simulink model "DiscCruiseController"  (Simulink 7.7)
settings: Solver=ode45  StartTime=0.0  StopTime=10.0  RelTol=1e-3
undefined symbols (not defined in the file): DT_Integrator, H, PID, suspension_lib, z
settings Model: Creator=jporter  LastModifiedBy=jporter

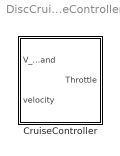
== system DiscCruiseController ==
  CruiseController : Subsystem

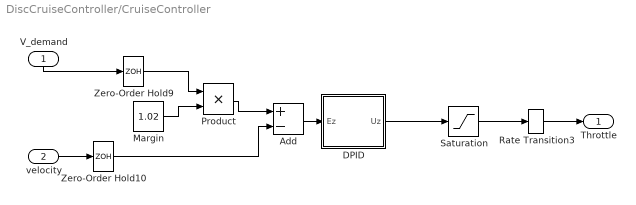
== system DiscCruiseController/CruiseController ==
  V_demand : Inport
  velocity : Inport  Port=2
  Add : Sum  Inputs=+-
  DPID : Subsystem  AncestorBlock=suspension_lib/PID:H(z)  mask{Ts=.1, K_P=7, K_D=0, tau_D=.1/pi, P_MAX=1500*2, P_MIN=-1500*2, X_DMAX=1500*2, X_DMIN=-1500*2, X_D0=0, K_I=0, X_IMAX=1500, X_IMIN=-1500, X_I0=0}
      mask prompts: Ts "Ts (seconds)"
  Margin : Constant  Value=1.02
  Product : Product  RndMeth=Zero
  Rate Transition3 : RateTransition  X0=1  OutPortSampleTime=0
  Saturation : Saturate  UpperLimit=1  LowerLimit=0
  Zero-Order Hold10 : ZeroOrderHold  Priority=-1  SampleTime=0.1
  Zero-Order Hold9 : ZeroOrderHold  Priority=-1  SampleTime=0.1
  Throttle : Outport
  wires:
  Product/1 -> Add/1
  Add/1 -> DPID/1(Ez)
  DPID/1(Uz) -> Saturation/1
  V_demand/1 -> Zero-Order Hold9/1
  velocity/1 -> Zero-Order Hold10/1
  Saturation/1 -> Rate Transition3/1
  Margin/1 -> Product/2
  Rate Transition3/1 -> Throttle/1
  Zero-Order Hold9/1 -> Product/1
  Zero-Order Hold10/1 -> Add/2

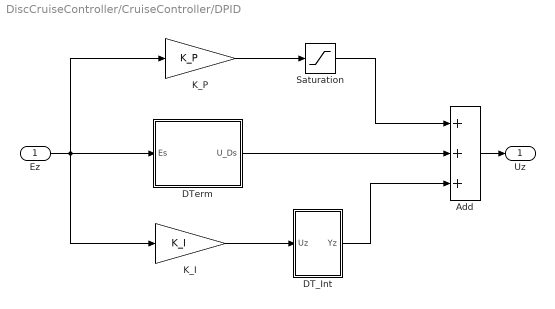
== system DiscCruiseController/CruiseController/DPID ==
  Ez : Inport
  Add : Sum  Inputs=+++
  DT_Int : Subsystem  AncestorBlock=suspension_lib/DT_Integrator  mask{Ts=Ts, X0=X_I0, X_MIN=X_IMIN, X_MAX=X_IMAX}
      mask prompts: Ts "Ts (seconds)"
  DTerm : Subsystem
  K_I : Gain  Gain=K_I
  K_P : Gain  Gain=K_P
  Saturation : Saturate  UpperLimit=P_MAX  LowerLimit=P_MIN
  Uz : Outport
  wires:
  Saturation/1 -> Add/1
  Add/1 -> Uz/1
  DTerm/1(U_Ds) -> Add/2
  DT_Int/1(Yz) -> Add/3
  K_I/1 -> DT_Int/1(Uz)
  K_P/1 -> Saturation/1
  Ez/1 -> DTerm/1(Es), K_I/1, K_P/1

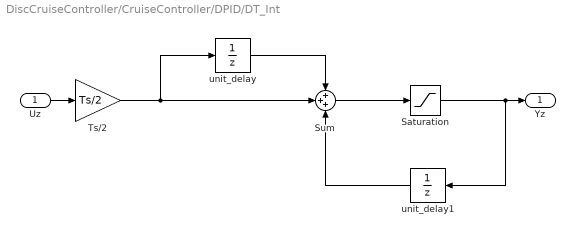
== system DiscCruiseController/CruiseController/DPID/DT_Int ==
  Uz : Inport
  Saturation : Saturate  UpperLimit=X_MAX  LowerLimit=X_MIN
  Sum : Sum  Inputs=+++
  Ts/2 : Gain  Gain=Ts/2
  unit_delay : UnitDelay  SampleTime=Ts
  unit_delay1 : UnitDelay  X0=X0  SampleTime=Ts
  Yz : Outport
  wires:
  unit_delay/1 -> Sum/1
  Sum/1 -> Saturation/1
  Saturation/1 -> unit_delay1/1, Yz/1
  unit_delay1/1 -> Sum/3
  Ts/2/1 -> unit_delay/1, Sum/2
  Uz/1 -> Ts/2/1

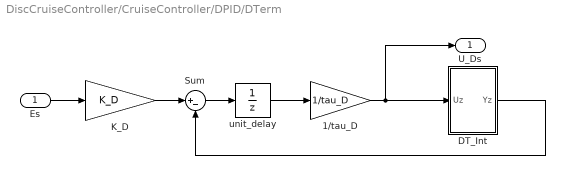
== system DiscCruiseController/CruiseController/DPID/DTerm ==
  Es : Inport
  1/tau_D : Gain  Gain=1/tau_D
  DT_Int : Subsystem  AncestorBlock=suspension_lib/DT_Integrator  mask{Ts=Ts, X0=X_D0, X_MIN=X_DMIN*tau_D, X_MAX=X_DMAX*tau_D}
      mask prompts: Ts "Ts (seconds)"
  K_D : Gain  Gain=K_D
  Sum : Sum  Inputs=|+-
  unit_delay : UnitDelay  SampleTime=Ts
  U_Ds : Outport
  wires:
  unit_delay/1 -> 1/tau_D/1
  Sum/1 -> unit_delay/1
  Es/1 -> K_D/1
  1/tau_D/1 -> U_Ds/1, DT_Int/1(Uz)
  DT_Int/1(Yz) -> Sum/2
  K_D/1 -> Sum/1

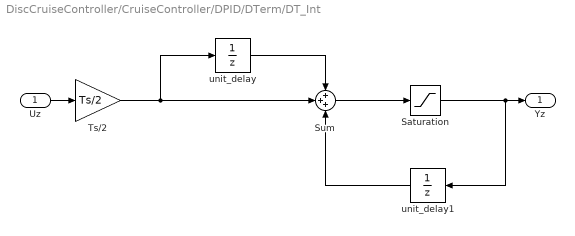
== system DiscCruiseController/CruiseController/DPID/DTerm/DT_Int ==
  Uz : Inport
  Saturation : Saturate  UpperLimit=X_MAX  LowerLimit=X_MIN
  Sum : Sum  Inputs=+++
  Ts/2 : Gain  Gain=Ts/2
  unit_delay : UnitDelay  SampleTime=Ts
  unit_delay1 : UnitDelay  X0=X0  SampleTime=Ts
  Yz : Outport
  wires:
  unit_delay/1 -> Sum/1
  Sum/1 -> Saturation/1
  Saturation/1 -> unit_delay1/1, Yz/1
  unit_delay1/1 -> Sum/3
  Ts/2/1 -> unit_delay/1, Sum/2
  Uz/1 -> Ts/2/1
